simulink model "full_maneuver_single_veh"  (R2020a)
settings: Solver=VariableStepAuto  StartTime=0.0  StopTime=90  FixedStep=0.1  MaxStep=5e-2  RelTol=1e-3
InitFcn:
  | totalVehicles = 5;
  | if exist('vehStatesBus', 'var')==0
  | load vehBuses
  | end
  | if exist('vehErrorsBus', 'var')==0
  | load vehBuses
  | end
libraries: simulink x69, powerlib_meascontrol x6, autolibshared x6, dspsigops x3, eeGeneralControl x2
(part 5 of 6)

== system full_maneuver_single_veh/Lo/Regular Vehicle Following/switch ==
  errors : Inport
  errorsDot : Inport  Port=2
  gap : Inport  Port=3
  h : Inport  Port=4
  d0 : Inport  Port=5
  vRef : Inport  Port=6
  Compare To Constant : simulink/Logic and Bit Operations/Compare To Constant  relop=<=  const=0  OutDataTypeStr=boolean
  Demux1 : Demux  Outputs=2
  Gain1 : Gain
  MATLAB Function : MATLAB Function  TreatAsAtomicUnit=on
  Scope : Scope  NumInputPorts=2
  Selector : Selector  InputPortWidth=2  IndexOptions=Index vector (dialog)  Indices=[2]  OutputSizes=1
  Sum2 : Sum  Inputs=+-
  inRange : Outport  VectorParamsAs1DForOutWhenUnconnected=off
  wires:
  Demux1/2 -> MATLAB Function/6(ea)
  Demux1/1 -> MATLAB Function/5(ehDot)
  errorsDot/1 -> Demux1/1
  MATLAB Function/1(maxGap) -> Sum2/2, Scope/2
  Gain1/1 -> MATLAB Function/1(h)
  Compare To Constant/1 -> inRange/1
  Selector/1 -> MATLAB Function/4(ev)
  Sum2/1 -> Compare To Constant/1
  gap/1 -> Sum2/1, Scope/1
  errors/1 -> Selector/1
  h/1 -> Gain1/1
  vRef/1 -> MATLAB Function/3(vRef)
  d0/1 -> MATLAB Function/2(d0)

== system full_maneuver_single_veh/Lo/findLeader/Subsystem ==
  ego : Inport
  all : Inport  Port=2
  Enable : EnablePort
  MATLAB Function : MATLAB Function  TreatAsAtomicUnit=on
  idx : Outport  InitialOutput=1  VectorParamsAs1DForOutWhenUnconnected=off
  wires:
  ego/1 -> MATLAB Function/1(ego)
  MATLAB Function/1(leaderIdx) -> idx/1
  all/1 -> MATLAB Function/2(allVehicles)

== system full_maneuver_single_veh/Lo/findLeader/farAwayVeh ==
  ego : Inport  OutDataTypeStr=Bus: vehStatesBus
  Bus Assignment : BusAssignment  AssignedSignals=X
  Bus Selector : BusSelector  OutputSignals=X
  Constant : Constant  Value=1000
  Sum : Sum  Inputs=|++
  Out1 : Outport  OutDataTypeStr=Bus: vehStatesBus  VectorParamsAs1DForOutWhenUnconnected=off
  wires:
  Sum/1 -> Bus Assignment/2  "X"
  Bus Selector/1 -> Sum/1  "<X>"
  Bus Assignment/1 -> Out1/1
  Constant/1 -> Sum/2
  ego/1 -> Bus Selector/1, Bus Assignment/1

== system full_maneuver_single_veh/p1/Find Leader/Subsystem ==
  ego : Inport
  all : Inport  Port=2
  Enable : EnablePort
  MATLAB Function : MATLAB Function  TreatAsAtomicUnit=on
  idx : Outport  InitialOutput=1  VectorParamsAs1DForOutWhenUnconnected=off
  wires:
  ego/1 -> MATLAB Function/1(ego)
  MATLAB Function/1(leaderIdx) -> idx/1
  all/1 -> MATLAB Function/2(allVehicles)

== system full_maneuver_single_veh/p1/Find Leader/farAwayVeh ==
  ego : Inport  OutDataTypeStr=Bus: vehStatesBus
  Bus Assignment : BusAssignment  AssignedSignals=X
  Bus Selector : BusSelector  OutputSignals=X
  Constant : Constant  Value=1000
  Sum : Sum  Inputs=|++
  Out1 : Outport  OutDataTypeStr=Bus: vehStatesBus  VectorParamsAs1DForOutWhenUnconnected=off
  wires:
  ego/1 -> Bus Assignment/1, Bus Selector/1
  Constant/1 -> Sum/2
  Bus Assignment/1 -> Out1/1
  Bus Selector/1 -> Sum/1  "<X>"
  Sum/1 -> Bus Assignment/2  "X"

== system full_maneuver_single_veh/p1/Lateral Control/Full State Observer ==
  note: yhat
  note: xhat
  measuredOutputs : Inport
  delta : Inport  Port=2
  Add1 : Sum  Inputs=|-+
  Gain : Gain  Gain=B  Multiplication=Matrix(K*u)
  Gain1 : Gain  Gain=C  Multiplication=Matrix(K*u)
  Gain2 : Gain  Gain=L  Multiplication=Matrix(K*u)
  Gain3 : Gain  Gain=A  Multiplication=Matrix(K*u)
  Integrator : Integrator  InitialCondition=[y0; 0; 0; 0]
  Signal Specification : SignalSpecification  Dimensions=[size(C,1) 1]
  Sum : Sum  Inputs=+++
  xhat : Outport  VectorParamsAs1DForOutWhenUnconnected=off
  wires:
  Gain2/1 -> Sum/1
  Signal Specification/1 -> Gain2/1
  Gain3/1 -> Sum/2
  Gain/1 -> Sum/3
  delta/1 -> Gain/1
  measuredOutputs/1 -> Add1/2
  Sum/1 -> Integrator/1
  Gain1/1 -> Add1/1
  Integrator/1 -> Gain1/1, Gain3/1, xhat/1
  Add1/1 -> Signal Specification/1

== system full_maneuver_single_veh/p1/Maneuver State/Triggered Subsystem ==
  Trigger : TriggerPort  VariantControl=Variant
  Constant : Constant  OutDataTypeStr=fixdt(1,16,0)
  Out1 : Outport  InitialOutput=0  VectorParamsAs1DForOutWhenUnconnected=off
  wires:
  Constant/1 -> Out1/1

== system full_maneuver_single_veh/p1/Maneuver State/Triggered Subsystem1 ==
  Trigger : TriggerPort  VariantControl=Variant
  Constant : Constant  Value=true  OutDataTypeStr=boolean
  Out1 : Outport  OutDataTypeStr=boolean  InitialOutput=0  VectorParamsAs1DForOutWhenUnconnected=off
  wires:
  Constant/1 -> Out1/1

== system full_maneuver_single_veh/p1/Maneuver State/safeErrors ==
  errors : Inport
  AND : Logic  Inputs=1  IconShape=distinctive  AllPortsSameDT=off  OutDataTypeStr=boolean
  Compare To Constant4 : simulink/Logic and Bit Operations/Compare To Constant  relop=>=  const=-0.1  OutDataTypeStr=boolean
  Memory : Memory
  Triggered Subsystem1 : Subsystem  TreatAsAtomicUnit=on
  safetyFlag : Outport  VectorParamsAs1DForOutWhenUnconnected=off
  wires:
  Compare To Constant4/1 -> AND/1
  AND/1 -> Triggered Subsystem1/Trigger
  errors/1 -> Compare To Constant4/1
  Triggered Subsystem1/1(Out1) -> Memory/1
  Memory/1 -> safetyFlag/1

== system full_maneuver_single_veh/p1/Maneuver State/safeErrors1 ==
  errors : Inport
  AND : Logic  Inputs=1  IconShape=distinctive  AllPortsSameDT=off  OutDataTypeStr=boolean
  Compare To Constant4 : simulink/Logic and Bit Operations/Compare To Constant  relop=>=  const=-0.1  OutDataTypeStr=boolean
  safetyFlag : Outport  VectorParamsAs1DForOutWhenUnconnected=off
  wires:
  Compare To Constant4/1 -> AND/1
  errors/1 -> Compare To Constant4/1
  AND/1 -> safetyFlag/1

== system full_maneuver_single_veh/p1/Maneuver State/safeErrors2 ==
  errors : Inport
  AND : Logic  Inputs=1  IconShape=distinctive  AllPortsSameDT=off  OutDataTypeStr=boolean
  Compare To Constant4 : simulink/Logic and Bit Operations/Compare To Constant  relop=>=  const=-0.1  OutDataTypeStr=boolean
  safetyFlag : Outport  VectorParamsAs1DForOutWhenUnconnected=off
  wires:
  Compare To Constant4/1 -> AND/1
  AND/1 -> safetyFlag/1
  errors/1 -> Compare To Constant4/1

== system full_maneuver_single_veh/p1/Maneuver State/steadyState ==
  u : Inport
  AND : Logic  Inputs=1  IconShape=distinctive  AllPortsSameDT=off  OutDataTypeStr=boolean
  Abs2 : Abs
  Compare To Constant2 : simulink/Logic and Bit Operations/Compare To Constant  relop=<=  const=0.2  OutDataTypeStr=boolean
  Mux : Mux  Inputs=2
  Transport Delay2 : TransportDelay
  ssFlag : Outport  VectorParamsAs1DForOutWhenUnconnected=off
  wires:
  Compare To Constant2/1 -> AND/1
  u/1 -> Transport Delay2/1, Mux/2
  Abs2/1 -> Compare To Constant2/1
  Transport Delay2/1 -> Mux/1
  AND/1 -> ssFlag/1
  Mux/1 -> Abs2/1

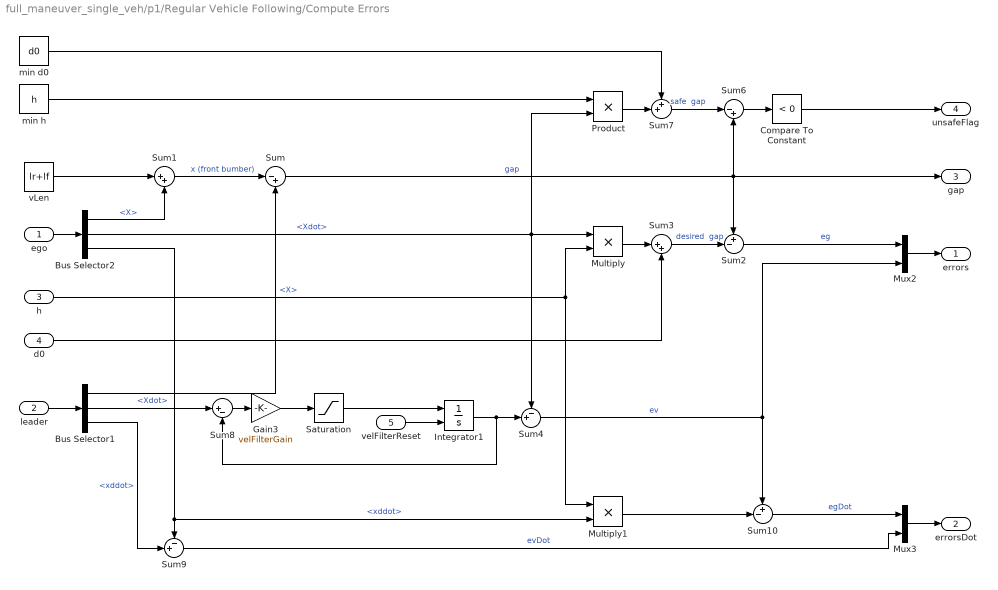
== system full_maneuver_single_veh/p1/Regular Vehicle Following/Compute Errors ==
  ego : Inport
  leader : Inport  Port=2
  h : Inport  Port=3
  d0 : Inport  Port=4
  velFilterReset : Inport  Port=5
  Bus Selector1 : BusSelector  OutputSignals=X,Xdot,xddot
  Bus Selector2 : BusSelector  OutputSignals=X,Xdot,xddot
  Compare To Constant : simulink/Logic and Bit Operations/Compare To Constant  relop=<  const=0  OutDataTypeStr=boolean
  Gain3 : Gain  Gain=velFilterGain
  Integrator1 : Integrator  ExternalReset=rising  InitialCondition=vx0
  Multiply : Product
  Multiply1 : Product
  Mux2 : Mux  Inputs=2
  Mux3 : Mux  Inputs=2
  Product : Product
  Saturation : Saturate  UpperLimit=maxAcceleration  LowerLimit=minAcceleration
  Sum : Sum  Inputs=|-+
  Sum1 : Sum  Inputs=|++
  Sum10 : Sum  Inputs=+-|
  Sum2 : Sum  Inputs=+-|
  Sum3 : Sum  Inputs=|++
  Sum4 : Sum  Inputs=-+|
  Sum6 : Sum  Inputs=|-+
  Sum7 : Sum  Inputs=++|
  Sum8 : Sum  Inputs=|+-
  Sum9 : Sum  Inputs=-+|
  min d0 : Constant  Value=d0
  min h : Constant  Value=h
  vLen : Constant  Value=lr+lf
  errors : Outport  VectorParamsAs1DForOutWhenUnconnected=off
  errorsDot : Outport  Port=2
  "gap " : Outport  Port=3  VectorParamsAs1DForOutWhenUnconnected=off
  unsafeFlag : Outport  Port=4  VectorParamsAs1DForOutWhenUnconnected=off
  wires:
  leader/1 -> Bus Selector1/1
  ego/1 -> Bus Selector2/1
  Mux3/1 -> errorsDot/1
  Sum9/1 -> Mux3/2  "evDot"
  Sum10/1 -> Mux3/1  "egDot"
  Multiply1/1 -> Sum10/2
  Bus Selector2/3 -> Multiply1/2, Sum9/1  "<xddot>"
  Bus Selector1/3 -> Sum9/2  "<xddot>"
  Sum8/1 -> Gain3/1
  Integrator1/1 -> Sum8/2, Sum4/2
  Saturation/1 -> Integrator1/1
  Gain3/1 -> Saturation/1
  Sum4/1 -> Sum10/1, Mux2/2  "ev"
  Bus Selector1/2 -> Sum8/1  "<Xdot>"
  h/1 -> Multiply1/1, Multiply/2
  Bus Selector2/1 -> Sum1/2  "<X>"
  Sum/1 -> "gap "/1, Sum6/2, Sum2/1  "gap"
  Multiply/1 -> Sum3/1
  min d0/1 -> Sum7/1
  vLen/1 -> Sum1/1
  d0/1 -> Sum3/2
  Bus Selector2/2 -> Product/2, Multiply/1, Sum4/1  "<Xdot>"
  Sum1/1 -> Sum/1  "x (front bumber)"
  Sum3/1 -> Sum2/2  "desired  gap"
  Product/1 -> Sum7/2
  Bus Selector1/1 -> Sum/2  "<X>"
  Sum2/1 -> Mux2/1  "eg"
  Compare To Constant/1 -> unsafeFlag/1
  min h/1 -> Product/1
  Sum7/1 -> Sum6/1  "safe  gap"
  Sum6/1 -> Compare To Constant/1
  velFilterReset/1 -> Integrator1/2
  Mux2/1 -> errors/1

== system full_maneuver_single_veh/p1/Regular Vehicle Following/Define Desired Distance ==
  extraSpaceFlag : Inport
  Constant : Constant  Value=h
  Constant1 : Constant  Value=d0
  Constant2 : Constant  Value=hLC
  Constant3 : Constant  Value=d0LC
  Demux : Demux  Outputs=2
  Integrator : Integrator  InitialCondition=[h d0]
  Mux : Mux  Inputs=2
  Mux1 : Mux  Inputs=2
  Saturation1 : Saturate  UpperLimit=hFilterSaturation/2  LowerLimit=-hFilterSaturation
  Sum5 : Sum  Inputs=|+-
  Switch : Switch  Criteria=u2 > Threshold
  hFilterGain : Gain  Gain=hFilterGain
  h : Outport
  d0 : Outport  Port=2
  wires:
  Demux/2 -> d0/1
  Demux/1 -> h/1
  Integrator/1 -> Sum5/2, Demux/1
  Saturation1/1 -> Integrator/1
  extraSpaceFlag/1 -> Switch/2
  Constant1/1 -> Mux/2
  Constant3/1 -> Mux1/2
  Switch/1 -> Sum5/1
  Mux1/1 -> Switch/1
  Sum5/1 -> hFilterGain/1
  Constant2/1 -> Mux1/1
  hFilterGain/1 -> Saturation1/1
  Constant/1 -> Mux/1
  Mux/1 -> Switch/3

== system full_maneuver_single_veh/p1/Regular Vehicle Following/Veh Following ==
  errors : Inport
  errorsDot : Inport  Port=2
  realInput : Inport  Port=3
  leaderChange : Inport  Port=4
  inRange : Inport  Port=5
  Demux : Demux  Outputs=2
  Demux1 : Demux  Outputs=2
  Gain : Gain  Gain=Ka
  Gain1 : Gain  Gain=Kdd
  Gain3 : Gain  Commented=on  Gain=10
  Integrator1 : Integrator  Commented=on  ExternalReset=either  InitialConditionSource=external  InitialCondition=vx0
  Kd : Gain  Gain=Kd
  Kp : Gain  Gain=Kp
  Saturation : Saturate  Commented=on  UpperLimit=maxComfAccel  LowerLimit=minAcceleration
  Saturation1 : Saturate  UpperLimit=maxGapError  LowerLimit=minGapError
  Scope : Scope  NumInputPorts=6
  Sum : Sum  Inputs=+-|
  Sum1 : Sum  Inputs=+++++
  Sum8 : Sum  Commented=on  Inputs=|+-
  Transport Delay : TransportDelay  DelayTime=0.1
  integralTerm : Subsystem
  u : Outport  VectorParamsAs1DForOutWhenUnconnected=off
  wires:
  Demux1/2 -> Gain/1  "evDot"
  Demux1/1 -> Gain1/1  "egDot"
  errorsDot/1 -> Demux1/1
  Sum1/1 -> u/1, Scope/6, Sum/1, Sum8/1
  Gain/1 -> Scope/5, Sum1/5
  Gain1/1 -> Scope/4, Sum1/4
  integralTerm/1(Out1) -> Transport Delay/1
  Sum/1 -> integralTerm/2(inputDiff)
  realInput/1 -> Integrator1/3, Sum/2
  Transport Delay/1 -> Scope/1, Sum1/1
  leaderChange/1 -> integralTerm/3(leaderChange)
  Demux/1 -> Saturation1/1  "eg"
  Kd/1 -> Scope/3, Sum1/3
  Demux/2 -> Kd/1  "ev"
  Saturation1/1 -> Kp/1, integralTerm/1(eh)
  errors/1 -> Demux/1
  Integrator1/1 -> Sum8/2
  Saturation/1 -> Integrator1/1
  Sum8/1 -> Gain3/1
  Gain3/1 -> Saturation/1
  Kp/1 -> Scope/2, Sum1/2
  inRange/1 -> Integrator1/2, integralTerm/Enable

== system full_maneuver_single_veh/p1/Regular Vehicle Following/Velocity Control ==
  ev : Inport
  ea : Inport  Port=2
  realInput : Inport  Port=3
  Abs : Abs
  Compare To Constant : simulink/Logic and Bit Operations/Compare To Constant  relop=<=  const=0.2  OutDataTypeStr=boolean
  Gain : Gain  Gain=velKd
  Scope : Scope  NumInputPorts=4
  Sum1 : Sum  Inputs=|-+
  Sum3 : Sum  Inputs=+++
  Transport Delay : TransportDelay  DelayTime=0.1
  integral term : Subsystem
  velKp : Gain  Gain=velKp
  u : Outport  VectorParamsAs1DForOutWhenUnconnected=off
  wires:
  Transport Delay/1 -> Sum1/2
  Compare To Constant/1 -> integral term/Enable
  integral term/1(Out1) -> Sum3/1, Scope/1
  Abs/1 -> Compare To Constant/1
  Sum1/1 -> Abs/1
  ev/1 -> velKp/1, integral term/1(ev)
  velKp/1 -> Scope/2, Sum3/2
  realInput/1 -> Sum1/1
  ea/1 -> Gain/1
  Gain/1 -> Scope/3, Sum3/3
  Sum3/1 -> u/1, Scope/4, Transport Delay/1

== system full_maneuver_single_veh/p1/Regular Vehicle Following/Velocity Error ==
  ego : Inport
  velRef : Inport  Port=2
  filterReset : Inport  Port=3
  Bus Selector : BusSelector  OutputSignals=Xdot,xddot
  Gain : Gain  Gain=-1
  Gain3 : Gain  Gain=velFilterGain
  Integrator1 : Integrator  ExternalReset=rising  InitialCondition=vx0
  NOT : Logic  Operator=NOT  IconShape=distinctive  AllPortsSameDT=off  OutDataTypeStr=boolean
  Saturation : Saturate  UpperLimit=maxComfAccel  LowerLimit=minComfAccel
  Sum : Sum  Inputs=+-|
  Sum8 : Sum  Inputs=|+-
  ev : Outport
  ea : Outport  Port=2
  wires:
  Sum8/1 -> Gain3/1
  Gain3/1 -> Saturation/1
  Saturation/1 -> Integrator1/1
  velRef/1 -> Sum8/1
  Integrator1/1 -> Sum/1, Sum8/2
  ego/1 -> Bus Selector/1
  Bus Selector/1 -> Sum/2  "<Xdot>"
  Bus Selector/2 -> Gain/1  "<xddot>"
  Sum/1 -> ev/1
  Gain/1 -> ea/1
  filterReset/1 -> NOT/1
  NOT/1 -> Integrator1/2

== system full_maneuver_single_veh/p1/Regular Vehicle Following/switch free flow ==
  errors : Inport
  errorsDot : Inport  Port=2
  gap : Inport  Port=3
  h : Inport  Port=4
  d0 : Inport  Port=5
  vRef : Inport  Port=6
  Demux1 : Demux  Outputs=2
  Gain1 : Gain
  MATLAB Function : MATLAB Function  TreatAsAtomicUnit=on
  Relay : Relay  OnSwitchValue=1  OffSwitchValue=-1
  Scope : Scope  NumInputPorts=2
  Selector : Selector  InputPortWidth=2  IndexOptions=Index vector (dialog)  Indices=[2]  OutputSizes=1
  Sum2 : Sum  Inputs=-+
  inRange : Outport  VectorParamsAs1DForOutWhenUnconnected=off
  wires:
  Demux1/2 -> MATLAB Function/6(ea)
  Demux1/1 -> MATLAB Function/5(ehDot)
  errorsDot/1 -> Demux1/1
  MATLAB Function/1(maxGap) -> Sum2/2, Scope/2
  Gain1/1 -> MATLAB Function/1(h)
  Relay/1 -> inRange/1
  Selector/1 -> MATLAB Function/4(ev)
  Sum2/1 -> Relay/1
  gap/1 -> Sum2/1, Scope/1
  errors/1 -> Selector/1
  h/1 -> Gain1/1
  vRef/1 -> MATLAB Function/3(vRef)
  d0/1 -> MATLAB Function/2(d0)

== system full_maneuver_single_veh/p1/Virtual Vehicle Following/Compute Errors ==
  ego : Inport
  leader : Inport  Port=2
  h : Inport  Port=3
  d0 : Inport  Port=4
  velFilterReset : Inport  Port=5
  Bus Selector1 : BusSelector  OutputSignals=X,Xdot,xddot
  Bus Selector2 : BusSelector  OutputSignals=X,Xdot,xddot
  Compare To Constant : simulink/Logic and Bit Operations/Compare To Constant  relop=<  const=0  OutDataTypeStr=boolean
  Gain3 : Gain  Gain=velFilterGain
  Integrator1 : Integrator  ExternalReset=rising  InitialCondition=vx0
  Multiply : Product
  Multiply1 : Product
  Mux2 : Mux  Inputs=2
  Mux3 : Mux  Inputs=2
  Product : Product
  Saturation : Saturate  UpperLimit=maxAcceleration  LowerLimit=minAcceleration
  Sum : Sum  Inputs=|-+
  Sum1 : Sum  Inputs=|++
  Sum10 : Sum  Inputs=+-|
  Sum2 : Sum  Inputs=+-|
  Sum3 : Sum  Inputs=|++
  Sum4 : Sum  Inputs=-+|
  Sum6 : Sum  Inputs=|-+
  Sum7 : Sum  Inputs=++|
  Sum8 : Sum  Inputs=|+-
  Sum9 : Sum  Inputs=-+|
  min d0 : Constant  Value=d0
  min h : Constant  Value=h
  vLen : Constant  Value=lr+lf
  errors : Outport  VectorParamsAs1DForOutWhenUnconnected=off
  errorsDot : Outport  Port=2
  "gap " : Outport  Port=3  VectorParamsAs1DForOutWhenUnconnected=off
  unsafeFlag : Outport  Port=4  VectorParamsAs1DForOutWhenUnconnected=off
  wires:
  leader/1 -> Bus Selector1/1
  ego/1 -> Bus Selector2/1
  Mux3/1 -> errorsDot/1
  Sum9/1 -> Mux3/2  "evDot"
  Sum10/1 -> Mux3/1  "egDot"
  Multiply1/1 -> Sum10/2
  Bus Selector2/3 -> Multiply1/2, Sum9/1  "<xddot>"
  Bus Selector1/3 -> Sum9/2  "<xddot>"
  Sum8/1 -> Gain3/1
  Integrator1/1 -> Sum8/2, Sum4/2
  Saturation/1 -> Integrator1/1
  Gain3/1 -> Saturation/1
  Sum4/1 -> Sum10/1, Mux2/2  "ev"
  Bus Selector1/2 -> Sum8/1  "<Xdot>"
  h/1 -> Multiply1/1, Multiply/2
  Bus Selector2/1 -> Sum1/2  "<X>"
  Sum/1 -> Sum6/2, "gap "/1, Sum2/1  "gap"
  Multiply/1 -> Sum3/1
  min d0/1 -> Sum7/1
  vLen/1 -> Sum1/1
  d0/1 -> Sum3/2
  Bus Selector2/2 -> Product/2, Multiply/1, Sum4/1  "<Xdot>"
  Sum1/1 -> Sum/1  "x (front bumber)"
  Sum3/1 -> Sum2/2  "desired  gap"
  Product/1 -> Sum7/2
  Bus Selector1/1 -> Sum/2  "<X>"
  Sum2/1 -> Mux2/1  "eg"
  Compare To Constant/1 -> unsafeFlag/1
  min h/1 -> Product/1
  Sum7/1 -> Sum6/1  "safe  gap"
  Sum6/1 -> Compare To Constant/1
  velFilterReset/1 -> Integrator1/2
  Mux2/1 -> errors/1

== system full_maneuver_single_veh/p1/Virtual Vehicle Following/Define Desired Distance ==
  extraSpaceFlag : Inport
  Constant : Constant  Value=h
  Constant1 : Constant  Value=d0
  Constant2 : Constant  Value=hLC
  Constant3 : Constant  Value=d0LC
  Demux : Demux  Outputs=2
  Integrator : Integrator  InitialCondition=[h d0]
  Mux : Mux  Inputs=2
  Mux1 : Mux  Inputs=2
  Saturation1 : Saturate  UpperLimit=hFilterSaturation/2  LowerLimit=-hFilterSaturation
  Sum5 : Sum  Inputs=|+-
  Switch : Switch  Criteria=u2 > Threshold
  hFilterGain : Gain  Gain=hFilterGain
  h : Outport
  d0 : Outport  Port=2
  wires:
  Demux/2 -> d0/1
  Demux/1 -> h/1
  Integrator/1 -> Sum5/2, Demux/1
  Saturation1/1 -> Integrator/1
  extraSpaceFlag/1 -> Switch/2
  Constant1/1 -> Mux/2
  Constant3/1 -> Mux1/2
  Switch/1 -> Sum5/1
  Mux1/1 -> Switch/1
  Sum5/1 -> hFilterGain/1
  Constant2/1 -> Mux1/1
  hFilterGain/1 -> Saturation1/1
  Constant/1 -> Mux/1
  Mux/1 -> Switch/3

== system full_maneuver_single_veh/p1/Virtual Vehicle Following/Min Velocity Control ==
  ev : Inport
  ea : Inport  Port=2
  realInput : Inport  Port=3
  Abs : Abs
  Compare To Constant : simulink/Logic and Bit Operations/Compare To Constant  relop=<=  const=0.2  OutDataTypeStr=boolean
  Gain : Gain  Gain=velKd
  Scope : Scope  NumInputPorts=4
  Sum1 : Sum  Inputs=|-+
  Sum3 : Sum  Inputs=+++
  Transport Delay : TransportDelay  DelayTime=0.1
  integral term : Subsystem
  velKp : Gain  Gain=velKp
  u : Outport  VectorParamsAs1DForOutWhenUnconnected=off
  wires:
  Transport Delay/1 -> Sum1/2
  Compare To Constant/1 -> integral term/Enable
  integral term/1(Out1) -> Sum3/1, Scope/1
  Abs/1 -> Compare To Constant/1
  Sum1/1 -> Abs/1
  ev/1 -> velKp/1, integral term/1(ev)
  velKp/1 -> Scope/2, Sum3/2
  Sum3/1 -> Scope/4, Transport Delay/1, u/1
  realInput/1 -> Sum1/1
  ea/1 -> Gain/1
  Gain/1 -> Scope/3, Sum3/3

== system full_maneuver_single_veh/p1/Virtual Vehicle Following/Min Velocity Error ==
  ego : Inport
  velRef : Inport  Port=2
  filterReset : Inport  Port=3
  Bus Selector : BusSelector  OutputSignals=Xdot,xddot
  Gain : Gain  Gain=-1
  Gain3 : Gain  Gain=velFilterGain
  Integrator1 : Integrator  ExternalReset=rising  InitialCondition=vx0
  Saturation : Saturate  UpperLimit=maxComfAccel  LowerLimit=minComfAccel
  Sum : Sum  Inputs=+-|
  Sum8 : Sum  Inputs=|+-
  ev : Outport
  ea : Outport  Port=2
  wires:
  filterReset/1 -> Integrator1/2
  Gain/1 -> ea/1
  Sum/1 -> ev/1
  Bus Selector/2 -> Gain/1  "<xddot>"
  Bus Selector/1 -> Sum/2  "<Xdot>"
  ego/1 -> Bus Selector/1
  Integrator1/1 -> Sum8/2, Sum/1
  velRef/1 -> Sum8/1
  Saturation/1 -> Integrator1/1
  Gain3/1 -> Saturation/1
  Sum8/1 -> Gain3/1

== system full_maneuver_single_veh/p1/Virtual Vehicle Following/Virtual Leader Following ==
  errors : Inport
  errorsDot : Inport  Port=2
  realInput : Inport  Port=3
  leaderChange : Inport  Port=4
  inRange : Inport  Port=5
  Demux : Demux  Outputs=2
  Demux1 : Demux  Outputs=2
  Gain : Gain  Gain=10
  Gain3 : Gain  Gain=Ka
  Gain4 : Gain  Gain=Kdd
  Gain5 : Gain  Gain=10
  Integrator1 : Integrator  ExternalReset=rising  InitialConditionSource=external  InitialCondition=vx0
  Integrator2 : Integrator  ExternalReset=rising
  Kd : Gain  Gain=Kd
  Kp : Gain  Gain=Kp
  Saturation : Saturate  UpperLimit=maxComfAccel  LowerLimit=minAcceleration
  Saturation1 : Saturate  UpperLimit=maxGapError  LowerLimit=-maxGapError*2
  Scope : Scope  NumInputPorts=6
  Sum : Sum  Inputs=+-|
  Sum1 : Sum  Inputs=+++++
  Sum8 : Sum  Inputs=|+-
  Sum9 : Sum  Inputs=|+-
  Transport Delay : TransportDelay  DelayTime=0.1
  integralTerm : Subsystem
  u : Outport  VectorParamsAs1DForOutWhenUnconnected=off
  wires:
  errorsDot/1 -> Demux1/1
  errors/1 -> Demux/1
  Saturation1/1 -> Sum9/1
  Sum9/1 -> Gain/1
  Gain/1 -> Integrator2/1
  Demux/1 -> Saturation1/1
  Kd/1 -> Scope/3, Sum1/3
  Gain5/1 -> Saturation/1
  inRange/1 -> integralTerm/Enable, Integrator1/2
  Transport Delay/1 -> Scope/1, Sum1/1
  Integrator2/1 -> integralTerm/1(eh), Kp/1, Sum9/2
  Kp/1 -> Scope/2, Sum1/2
  Sum/1 -> integralTerm/2(inputDiff)
  Sum8/1 -> Gain5/1
  realInput/1 -> Integrator1/3, Sum/2
  Gain4/1 -> Scope/4, Sum1/4
  Saturation/1 -> Integrator1/1
  Demux/2 -> Kd/1  "ev"
  Gain3/1 -> Scope/5, Sum1/5
  Integrator1/1 -> u/1, Sum8/2
  Sum1/1 -> Sum/1, Scope/6, Sum8/1
  integralTerm/1(Out1) -> Transport Delay/1
  leaderChange/1 -> Integrator2/2, integralTerm/3(leaderChange)
  Demux1/1 -> Gain4/1  "egDot"
  Demux1/2 -> Gain3/1  "evDot"

== system full_maneuver_single_veh/p1/Virtual Vehicle Following/switch min vel ==
  errors : Inport
  errorsDot : Inport  Port=2
  gap : Inport  Port=3
  h : Inport  Port=4
  d0 : Inport  Port=5
  vRef : Inport  Port=6
  Demux1 : Demux  Outputs=2
  Gain1 : Gain
  MATLAB Function : MATLAB Function  TreatAsAtomicUnit=on
  Relay1 : Relay  OnSwitchValue=1  OffSwitchValue=-1
  Scope : Scope  NumInputPorts=2
  Scope1 : Scope  NumInputPorts=2
  Selector : Selector  InputPortWidth=2  IndexOptions=Index vector (dialog)  Indices=[2]  OutputSizes=1
  Sum2 : Sum  Inputs=-+
  inRange : Outport  VectorParamsAs1DForOutWhenUnconnected=off
  wires:
  Demux1/2 -> MATLAB Function/6(ea)
  Demux1/1 -> MATLAB Function/5(ehDot)
  errorsDot/1 -> Demux1/1
  MATLAB Function/1(maxGap) -> Sum2/2, Scope/2
  Gain1/1 -> MATLAB Function/1(h)
  Relay1/1 -> Scope1/2, inRange/1
  Selector/1 -> MATLAB Function/4(ev)
  Sum2/1 -> Relay1/1, Scope1/1
  gap/1 -> Sum2/1, Scope/1
  errors/1 -> Selector/1
  h/1 -> Gain1/1
  vRef/1 -> MATLAB Function/3(vRef)
  d0/1 -> MATLAB Function/2(d0)

== system full_maneuver_single_veh/Fd/Maneuver State/safeErrors/Triggered Subsystem1 ==
  Trigger : TriggerPort  VariantControl=Variant
  Constant : Constant  Value=true  OutDataTypeStr=boolean
  Out1 : Outport  OutDataTypeStr=boolean  InitialOutput=0  VectorParamsAs1DForOutWhenUnconnected=off
  wires:
  Constant/1 -> Out1/1

== system full_maneuver_single_veh/Fd/Regular Vehicle Following/Veh Following/integralTerm ==
  eh : Inport
  inputDiff : Inport  Port=2
  leaderChange : Inport  Port=3
  Enable : EnablePort  ShowOutputPort=on
  Anti-windup gain : Gain  Gain=sqrt(Ki/Kd)
  Integrator : Integrator  ExternalReset=either
  Ki : Gain  Gain=Ki
  Scope : Scope  NumInputPorts=2
  Sum5 : Sum  Inputs=-+|
  XOR : Logic  Operator=XOR  IconShape=distinctive  AllPortsSameDT=off  OutDataTypeStr=boolean
  Out1 : Outport  OutputWhenDisabled=reset  InitialOutput=0  VectorParamsAs1DForOutWhenUnconnected=off
  wires:
  eh/1 -> Ki/1
  Integrator/1 -> Out1/1
  XOR/1 -> Integrator/2
  leaderChange/1 -> XOR/1
  Enable/1 -> XOR/2
  Sum5/1 -> Integrator/1, Scope/2
  Ki/1 -> Sum5/2
  Anti-windup gain/1 -> Sum5/1, Scope/1
  inputDiff/1 -> Anti-windup gain/1

== system full_maneuver_single_veh/Fd/Regular Vehicle Following/Velocity Control/integral term ==
  ev : Inport
  Enable : EnablePort  StatesWhenEnabling=reset
  Integrator2 : Integrator
  velKi : Gain  Gain=velKi
  Out1 : Outport  OutputWhenDisabled=reset  InitialOutput=0
  wires:
  velKi/1 -> Integrator2/1
  Integrator2/1 -> Out1/1
  ev/1 -> velKi/1

== system full_maneuver_single_veh/Fd/Virtual Vehicle Following/Min Velocity Control/integral term ==
  ev : Inport
  Enable : EnablePort  StatesWhenEnabling=reset
  Integrator2 : Integrator
  velKi : Gain  Gain=velKi
  Out1 : Outport  OutputWhenDisabled=reset  InitialOutput=0
  wires:
  velKi/1 -> Integrator2/1
  Integrator2/1 -> Out1/1
  ev/1 -> velKi/1

== system full_maneuver_single_veh/Fd/Virtual Vehicle Following/Virtual Leader Following/integralTerm ==
  eh : Inport
  inputDiff : Inport  Port=2
  leaderChange : Inport  Port=3
  Enable : EnablePort  ShowOutputPort=on
  Anti-windup gain : Gain  Gain=sqrt(Ki/Kd)
  Integrator : Integrator  ExternalReset=either
  Ki : Gain  Gain=Ki
  Scope : Scope  NumInputPorts=2
  Sum5 : Sum  Inputs=-+|
  XOR : Logic  Operator=XOR  IconShape=distinctive  AllPortsSameDT=off  OutDataTypeStr=boolean
  Out1 : Outport  OutputWhenDisabled=reset  InitialOutput=0  VectorParamsAs1DForOutWhenUnconnected=off
  wires:
  eh/1 -> Ki/1
  Integrator/1 -> Out1/1
  XOR/1 -> Integrator/2
  leaderChange/1 -> XOR/1
  Enable/1 -> XOR/2
  Sum5/1 -> Integrator/1, Scope/2
  Ki/1 -> Sum5/2
  Anti-windup gain/1 -> Sum5/1, Scope/1
  inputDiff/1 -> Anti-windup gain/1

== system full_maneuver_single_veh/Fd_bkp/Maneuver State/safeErrors/Triggered Subsystem1 ==
  Trigger : TriggerPort  VariantControl=Variant
  Constant : Constant  Value=true  OutDataTypeStr=boolean
  Out1 : Outport  OutDataTypeStr=boolean  InitialOutput=0  VectorParamsAs1DForOutWhenUnconnected=off
  wires:
  Constant/1 -> Out1/1

== system full_maneuver_single_veh/Fd_bkp/Regular Vehicle Following/Veh Following/integralTerm ==
  eh : Inport
  leaderChange : Inport  Port=2
  inputDiff : Inport  Port=3
  Enable : EnablePort  ShowOutputPort=on
  Anti-windup gain : Gain  Gain=sqrt(Ki/Kd)
  Integrator : Integrator  ExternalReset=rising
  Ki : Gain  Gain=Ki
  Sum5 : Sum  Inputs=-+|
  XOR : Logic  Operator=XOR  IconShape=distinctive  AllPortsSameDT=off  OutDataTypeStr=boolean
  Out1 : Outport  OutputWhenDisabled=reset  InitialOutput=0  VectorParamsAs1DForOutWhenUnconnected=off
  wires:
  eh/1 -> Ki/1
  Integrator/1 -> Out1/1
  XOR/1 -> Integrator/2
  leaderChange/1 -> XOR/1
  Enable/1 -> XOR/2
  Sum5/1 -> Integrator/1
  Ki/1 -> Sum5/2
  Anti-windup gain/1 -> Sum5/1
  inputDiff/1 -> Anti-windup gain/1

== system full_maneuver_single_veh/Fd_bkp/Regular Vehicle Following/Velocity Control/integral term ==
  ev : Inport
  Enable : EnablePort  StatesWhenEnabling=reset
  Integrator2 : Integrator
  velKi : Gain  Gain=velKi
  Out1 : Outport  OutputWhenDisabled=reset  InitialOutput=0
  wires:
  velKi/1 -> Integrator2/1
  Integrator2/1 -> Out1/1
  ev/1 -> velKi/1

== system full_maneuver_single_veh/Fd_bkp/Virtual Vehicle Following/Velocity Control1/integral term ==
  ev : Inport
  Enable : EnablePort  StatesWhenEnabling=reset
  Integrator2 : Integrator
  velKi : Gain  Gain=velKi
  Out1 : Outport  OutputWhenDisabled=reset  InitialOutput=0
  wires:
  velKi/1 -> Integrator2/1
  Integrator2/1 -> Out1/1
  ev/1 -> velKi/1

== system full_maneuver_single_veh/Fd_bkp/Virtual Vehicle Following/Velocity Control2/integral term ==
  ev : Inport
  Enable : EnablePort  StatesWhenEnabling=reset
  Integrator2 : Integrator
  velKi : Gain  Gain=velKi
  Out1 : Outport  OutputWhenDisabled=reset  InitialOutput=0
  wires:
  ev/1 -> velKi/1
  Integrator2/1 -> Out1/1
  velKi/1 -> Integrator2/1

== system full_maneuver_single_veh/Fd_bkp/Virtual Vehicle Following/Virtual Leader Following/integralTerm ==
  eh : Inport
  leaderChange : Inport  Port=2
  inputDiff : Inport  Port=3
  Enable : EnablePort  ShowOutputPort=on
  Anti-windup gain : Gain  Gain=sqrt(Ki/Kd)
  Integrator : Integrator  ExternalReset=rising
  Ki : Gain  Gain=Ki
  Sum5 : Sum  Inputs=-+|
  XOR : Logic  Operator=XOR  IconShape=distinctive  AllPortsSameDT=off  OutDataTypeStr=boolean
  Out1 : Outport  OutputWhenDisabled=reset  InitialOutput=0  VectorParamsAs1DForOutWhenUnconnected=off
  wires:
  eh/1 -> Ki/1
  Integrator/1 -> Out1/1
  XOR/1 -> Integrator/2
  leaderChange/1 -> XOR/1
  Enable/1 -> XOR/2
  Sum5/1 -> Integrator/1
  Ki/1 -> Sum5/2
  Anti-windup gain/1 -> Sum5/1
  inputDiff/1 -> Anti-windup gain/1

== system full_maneuver_single_veh/Fo/Regular Vehicle Following/Veh Following/integralTerm ==
  eh : Inport
  inputDiff : Inport  Port=2
  leaderChange : Inport  Port=3
  Enable : EnablePort  ShowOutputPort=on
  Anti-windup gain : Gain  Gain=sqrt(Ki/Kd)
  Integrator : Integrator  ExternalReset=either
  Ki : Gain  Gain=Ki
  Sum5 : Sum  Inputs=-+|
  XOR : Logic  Operator=XOR  IconShape=distinctive  AllPortsSameDT=off  OutDataTypeStr=boolean
  Out1 : Outport  OutputWhenDisabled=reset  InitialOutput=0  VectorParamsAs1DForOutWhenUnconnected=off
  wires:
  eh/1 -> Ki/1
  Integrator/1 -> Out1/1
  XOR/1 -> Integrator/2
  leaderChange/1 -> XOR/1
  Enable/1 -> XOR/2
  Sum5/1 -> Integrator/1
  Ki/1 -> Sum5/2
  Anti-windup gain/1 -> Sum5/1
  inputDiff/1 -> Anti-windup gain/1

== system full_maneuver_single_veh/Fo/Regular Vehicle Following/Velocity Control/integral term ==
  ev : Inport
  Enable : EnablePort  StatesWhenEnabling=reset
  Integrator2 : Integrator
  velKi : Gain  Gain=velKi
  Out1 : Outport  OutputWhenDisabled=reset  InitialOutput=0
  wires:
  velKi/1 -> Integrator2/1
  Integrator2/1 -> Out1/1
  ev/1 -> velKi/1

== system full_maneuver_single_veh/Ld/Regular Vehicle Following/Veh Following/integralTerm ==
  eh : Inport
  inputDiff : Inport  Port=2
  leaderChange : Inport  Port=3
  Enable : EnablePort  ShowOutputPort=on
  Anti-windup gain : Gain  Gain=sqrt(Ki/Kd)
  Integrator : Integrator  ExternalReset=either
  Ki : Gain  Gain=Ki
  Sum5 : Sum  Inputs=-+|
  XOR : Logic  Operator=XOR  IconShape=distinctive  AllPortsSameDT=off  OutDataTypeStr=boolean
  Out1 : Outport  OutputWhenDisabled=reset  InitialOutput=0  VectorParamsAs1DForOutWhenUnconnected=off
  wires:
  eh/1 -> Ki/1
  Integrator/1 -> Out1/1
  XOR/1 -> Integrator/2
  leaderChange/1 -> XOR/1
  Enable/1 -> XOR/2
  Sum5/1 -> Integrator/1
  Ki/1 -> Sum5/2
  Anti-windup gain/1 -> Sum5/1
  inputDiff/1 -> Anti-windup gain/1

== system full_maneuver_single_veh/Ld/Regular Vehicle Following/Velocity Control/integral term ==
  ev : Inport
  Enable : EnablePort  StatesWhenEnabling=reset
  Integrator2 : Integrator
  velKi : Gain  Gain=velKi
  Out1 : Outport  OutputWhenDisabled=reset  InitialOutput=0
  wires:
  velKi/1 -> Integrator2/1
  Integrator2/1 -> Out1/1
  ev/1 -> velKi/1

== system full_maneuver_single_veh/Lo/Regular Vehicle Following/Veh Following/integralTerm ==
  eh : Inport
  inputDiff : Inport  Port=2
  leaderChange : Inport  Port=3
  Enable : EnablePort  ShowOutputPort=on
  Anti-windup gain : Gain  Gain=sqrt(Ki/Kd)
  Integrator : Integrator  ExternalReset=either
  Ki : Gain  Gain=Ki
  Sum5 : Sum  Inputs=-+|
  XOR : Logic  Operator=XOR  IconShape=distinctive  AllPortsSameDT=off  OutDataTypeStr=boolean
  Out1 : Outport  OutputWhenDisabled=reset  InitialOutput=0  VectorParamsAs1DForOutWhenUnconnected=off
  wires:
  inputDiff/1 -> Anti-windup gain/1
  Anti-windup gain/1 -> Sum5/1
  Ki/1 -> Sum5/2
  Sum5/1 -> Integrator/1
  Enable/1 -> XOR/2
  leaderChange/1 -> XOR/1
  XOR/1 -> Integrator/2
  Integrator/1 -> Out1/1
  eh/1 -> Ki/1

== system full_maneuver_single_veh/Lo/Regular Vehicle Following/Velocity Control/integral term ==
  ev : Inport
  Enable : EnablePort  StatesWhenEnabling=reset
  Integrator2 : Integrator
  velKi : Gain  Gain=velKi
  Out1 : Outport  OutputWhenDisabled=reset  InitialOutput=0
  wires:
  ev/1 -> velKi/1
  Integrator2/1 -> Out1/1
  velKi/1 -> Integrator2/1

== system full_maneuver_single_veh/p1/Maneuver State/safeErrors/Triggered Subsystem1 ==
  Trigger : TriggerPort  VariantControl=Variant
  Constant : Constant  Value=true  OutDataTypeStr=boolean
  Out1 : Outport  OutDataTypeStr=boolean  InitialOutput=0  VectorParamsAs1DForOutWhenUnconnected=off
  wires:
  Constant/1 -> Out1/1

== system full_maneuver_single_veh/p1/Regular Vehicle Following/Veh Following/integralTerm ==
  eh : Inport
  inputDiff : Inport  Port=2
  leaderChange : Inport  Port=3
  Enable : EnablePort  ShowOutputPort=on
  Anti-windup gain : Gain  Gain=sqrt(Ki/Kd)
  Integrator : Integrator  ExternalReset=either
  Ki : Gain  Gain=Ki
  Scope : Scope  NumInputPorts=2
  Sum5 : Sum  Inputs=-+|
  XOR : Logic  Operator=XOR  IconShape=distinctive  AllPortsSameDT=off  OutDataTypeStr=boolean
  Out1 : Outport  OutputWhenDisabled=reset  InitialOutput=0  VectorParamsAs1DForOutWhenUnconnected=off
  wires:
  inputDiff/1 -> Anti-windup gain/1
  Anti-windup gain/1 -> Scope/1, Sum5/1
  Ki/1 -> Sum5/2
  Sum5/1 -> Scope/2, Integrator/1
  Enable/1 -> XOR/2
  leaderChange/1 -> XOR/1
  XOR/1 -> Integrator/2
  Integrator/1 -> Out1/1
  eh/1 -> Ki/1

== system full_maneuver_single_veh/p1/Regular Vehicle Following/Velocity Control/integral term ==
  ev : Inport
  Enable : EnablePort  StatesWhenEnabling=reset
  Integrator2 : Integrator
  velKi : Gain  Gain=velKi
  Out1 : Outport  OutputWhenDisabled=reset  InitialOutput=0
  wires:
  ev/1 -> velKi/1
  Integrator2/1 -> Out1/1
  velKi/1 -> Integrator2/1

== system full_maneuver_single_veh/p1/Virtual Vehicle Following/Min Velocity Control/integral term ==
  ev : Inport
  Enable : EnablePort  StatesWhenEnabling=reset
  Integrator2 : Integrator
  velKi : Gain  Gain=velKi
  Out1 : Outport  OutputWhenDisabled=reset  InitialOutput=0
  wires:
  ev/1 -> velKi/1
  Integrator2/1 -> Out1/1
  velKi/1 -> Integrator2/1

== system full_maneuver_single_veh/p1/Virtual Vehicle Following/Virtual Leader Following/integralTerm ==
  eh : Inport
  inputDiff : Inport  Port=2
  leaderChange : Inport  Port=3
  Enable : EnablePort  ShowOutputPort=on
  Anti-windup gain : Gain  Gain=sqrt(Ki/Kd)
  Integrator : Integrator  ExternalReset=either
  Ki : Gain  Gain=Ki
  Scope : Scope  NumInputPorts=2
  Sum5 : Sum  Inputs=-+|
  XOR : Logic  Operator=XOR  IconShape=distinctive  AllPortsSameDT=off  OutDataTypeStr=boolean
  Out1 : Outport  OutputWhenDisabled=reset  InitialOutput=0  VectorParamsAs1DForOutWhenUnconnected=off
  wires:
  inputDiff/1 -> Anti-windup gain/1
  Anti-windup gain/1 -> Scope/1, Sum5/1
  Ki/1 -> Sum5/2
  Sum5/1 -> Scope/2, Integrator/1
  Enable/1 -> XOR/2
  leaderChange/1 -> XOR/1
  XOR/1 -> Integrator/2
  Integrator/1 -> Out1/1
  eh/1 -> Ki/1

== matlab function full_maneuver_single_veh/Fd_bkp/Regular Vehicle Following/switch free flow/MATLAB Function ==
  data: h input; maxGap output; d0 input; vRef input; ev input; ehDot input; ea input; Kp parameter; Kd parameter; Ka parameter; Kdd parameter
function maxGap = followingGapThreshold(h, d0, vRef, ev, ehDot, ea, Kp, Kd, Ka, Kdd)

maxGap = h*vRef + d0 - 1/Kp*(Kd*ev + Kdd*ehDot + Ka*ea);

== matlab function full_maneuver_single_veh/Fd_bkp/Virtual Follower Manager/determineVirtualFollower ==
  data: nVehicles input; posInPlatoon input; lcStrategy input; virtualFollowerIdx output
function virtualFollowerIdx  = ...
    determineVirtualFollower(nVehicles, posInPlatoon, lcStrategy)

% Important assumption:
% The array of vehicles is ordered as [Ld, Fd, Lo, p1, ..., pN, Fo]

% To consider: would it be more organized to have two vehicle arrays (one 
% for each lane)?

switch lcStrategy
    case {1, 2} % synchronous, leader changes first
        virtualFollowerIdx = 2;
    case 3 % last veh changes first
        if posInPlatoon == nVehicles-4
            virtualFollowerIdx = 2;
        else
            virtualFollowerIdx = 3 + (posInPlatoon + 1);
        end
    otherwise
        error('[determineVirtualFollower in Simulink model] Unknown lane changing strategy]')
end

end

== matlab function full_maneuver_single_veh/Fd_bkp/Virtual Leader Manager/determineVirtualLeader ==
  data: nVehicles input; lcFlag input; lcDone input; virtualLeaderIdx output; posInPlatoon input; lcStrategy input
function virtualLeaderIdx  = ...
    determineVirtualLeader(nVehicles, lcFlag, lcDone, posInPlatoon, lcStrategy)

% Important assumption:
% The array of vehicles is ordered as [Ld, Fd, Lo, p1, ..., pN, Fo]

% To consider: would it be more organized to have two vehicle arrays (one 
% for each lane)?

if ~lcFlag% gap generating vehicle
    virtualLeaderIdx = nVehicles-1; % last platoon vehicle
    
else % lane changing vehicle
    switch lcStrategy
        case {1, 2} % synchronous, leader changes first
            if posInPlatoon == 1
                virtualLeaderIdx = 1;
            else
                virtualLeaderIdx = 3 + (posInPlatoon - 1);
            end
            
        case 3 % last veh changes first
            if ~lcDone
                virtualLeaderIdx = 1;
            else
                if posInPlatoon == 1
                    virtualLeaderIdx = 1;
                else
                    virtualLeaderIdx = 3 + (posInPlatoon - 1);
                end
            end
            
        otherwise
            error('[determineVirtualLeader in Simulink model] Unknown lane changing strategy]')
    end
end

end

== stateflow chart full_maneuver_single_veh/Fd_bkp/Virtual Vehicle Following/Chart ==
  state SpeedControlFreeFlow
    entry:
    state=2;
    during:
    u = uFreeFlowVelControl;
  state VehFollowing
    entry:
    state=0;
    during:
    u = uVehFoll;
  state SpeedControlMin
    entry:
    state = 1;
    during:
    u = uMinVelControl;
  state LogicError
    entry:
    state=-1;
  (default) -> VehFollowing
  VehFollowing -> SpeedControlFreeFlow [order 2] : [~leaderInRange]
  SpeedControlFreeFlow -> VehFollowing [order 1] : [leaderInRange]
  VehFollowing -> SpeedControlMin [order 1] : [~leaderInRangeBehind]
  SpeedControlMin -> VehFollowing [order 1] : [leaderInRangeBehind]
  LogicError -> VehFollowing
  SpeedControlFreeFlow -> LogicError [order 2] : [~leaderInRangeBehind]
  SpeedControlMin -> LogicError [order 2] : [~leaderInRange]
  data: uVehFoll input size=1; leaderInRange input; leaderInRangeBehind input size=1; uFreeFlowVelControl input; state output size=1; u output size=1; uMinVelControl input double

== matlab function full_maneuver_single_veh/Fd_bkp/Virtual Vehicle Following/switch free flow/MATLAB Function ==
  data: h input; maxGap output; d0 input; vRef input; ev input; ehDot input; ea input; Kp parameter; Kd parameter; Ka parameter; Kdd parameter
function maxGap = followingGapThreshold(h, d0, vRef, ev, ehDot, ea, Kp, Kd, Ka, Kdd)

maxGap = h*vRef + d0 - 1/Kp*(Kd*ev + Kdd*ehDot + Ka*ea);

== matlab function full_maneuver_single_veh/Fd_bkp/Virtual Vehicle Following/switch min vel/MATLAB Function ==
  data: h input; maxGap output; d0 input; vRef input; ev input; ehDot input; ea input; Kp parameter; Kd parameter; Ka parameter; Kdd parameter
function maxGap = followingGapThreshold(h, d0, vRef, ev, ehDot, ea, Kp, Kd, Ka, Kdd)

maxGap = h*vRef + d0 - 1/Kp*(Kd*ev + Kdd*ehDot + Ka*ea);

== stateflow chart full_maneuver_single_veh/p1/ControlChoice ==
  state RegVehFoll
    entry:
    state = 0;
    during:
    u = regFollInput;
  state AdjForLaneChange
    during:
    %if ~xor(leaderInRange, vLeaderInRange)
    state = 1;
    u = min(regFollInput, virtualFollInput);
    %elseif vLeaderInRange
    %    state = 2;
    %    u = virtualFollInput;
    %else
    %    state = 3;
    %    u = regFollInput;
    %end
  (default) -> RegVehFoll
  AdjForLaneChange -> RegVehFoll : [~vLeaderAssigned]
  RegVehFoll -> AdjForLaneChange : [startAdj && vLeaderAssigned]
  data: startAdj input; vLeaderAssigned input; regFollInput input; u output; virtualFollInput input; state output

== matlab function full_maneuver_single_veh/p1/Find Leader/Subsystem/MATLAB Function ==
  data: ego input Bus: vehStatesBus; allVehicles input; leaderIdx output
function leaderIdx  = findLeader(ego, allVehicles)

nv = length(allVehicles);

leaderIdx = nv+1;

farAwayVehicle.X = ego.X + 10^4;
farAwayVehicle.Y = ego.Y;
farAwayVehicle.Xdot = ego.Xdot;
farAwayVehicle.u = 0;

leader = farAwayVehicle;
% For non lane changing vehicles, the leader is whoever is longitudinally
% closer and with any part of the body in the same lane.
% 1.8m (half lane) + 0.9m (half veh width)
for n = 1:nv
    if allVehicles(n).X>ego.X
        if abs(allVehicles(n).Y - ego.Y)<=2.7 && allVehicles(n).X<leader.X
            leaderIdx = n;
        end
    end
end

== matlab function full_maneuver_single_veh/p1/Platoon Gap Generation Management/assignExtraSpace ==
  data: strategy input; extraSpaceFlag output; posInPlatoon input; platoonState input
function extraSpaceFlag = assignExtraSpace(strategy, posInPlatoon, platoonState)

myState = platoonState(posInPlatoon);

%%% Single vehicle case %%%
if length(platoonState)==1 
    extraSpaceFlag = myState<5;
    return
end

%%% Platoon case %%%
switch strategy
    case {1, 2}
        if posInPlatoon == 1
            followerState = platoonState(posInPlatoon+1);
            extraSpaceFlag = myState<5 || followerState<6; %any(platoonState<5)
        elseif posInPlatoon == length(platoonState)
            leaderState = platoonState(posInPlatoon-1);
            extraSpaceFlag = leaderState>1 && myState<5;
        else
            leaderState = platoonState(posInPlatoon-1);
            followerState = platoonState(posInPlatoon+1);
            extraSpaceFlag = leaderState>1 && (myState<5 || followerState<6);
        end
%     case 2
%         if posInPlatoon == 1
%             extraSpaceFlag = true;
%         else
%             extraSpaceFlag = platoonState(posInPlatoon-1)>5;
%         end
    case 3
        if posInPlatoon == length(platoonState)
            extraSpaceFlag = myState<5 || platoonState(1)<5;%any(platoonState<5)
            % eventually try platoonState(end-1)<5
        else
           followerState = platoonState(posInPlatoon+1); 
           extraSpaceFlag = followerState>4 && (myState<5 || followerState<6);
        end 
    otherwise
        error('Unknown strategy')
end

== matlab function full_maneuver_single_veh/p1/Platoon Gap Generation Management/assignvirtualLeader ==
  data: strategy input; virtualLeaderFlag output; posInPlatoon input; platoonState input
function virtualLeaderFlag = assignVirtualLeader(strategy, posInPlatoon, platoonState)

myState = platoonState(posInPlatoon);

%%% Single vehicle case %%%
if length(platoonState)==1 
    virtualLeaderFlag = myState<5;
    return
end

%%% Platoon case %%%
switch strategy
    case {1, 2}
        if posInPlatoon == 1
            virtualLeaderFlag = myState<5;
        else
            leaderState = platoonState(posInPlatoon-1);
            virtualLeaderFlag = leaderState>3 && myState<5 ;
        end
    case 3
        if posInPlatoon == 1
           followerState = platoonState(posInPlatoon+1);
           virtualLeaderFlag = followerState>4 && (myState<5 || followerState<6);
        elseif posInPlatoon == length(platoonState)
            leaderState = platoonState(posInPlatoon-1);
            virtualLeaderFlag = myState<5 || leaderState<5;
            % first condition is redundant since leaderState won't change
            % if myState<5 - leaving it there for clarity and completeness
        else
           leaderState = platoonState(posInPlatoon-1); 
           followerState = platoonState(posInPlatoon+1);
           virtualLeaderFlag = followerState>4 && (myState<5 || leaderState<5);
        end 
    otherwise
        error('Unknown strategy')
end

== matlab function full_maneuver_single_veh/p1/Regular Vehicle Following/switch free flow/MATLAB Function ==
  data: h input; maxGap output; d0 input; vRef input; ev input; ehDot input; ea input; Kp parameter; Kd parameter; Ka parameter; Kdd parameter
function maxGap = followingGapThreshold(h, d0, vRef, ev, ehDot, ea, Kp, Kd, Ka, Kdd)

maxGap = h*vRef + d0 - 1/Kp*(Kd*ev + Kdd*ehDot + Ka*ea);

== matlab function full_maneuver_single_veh/Lo/Regular Vehicle Following/switch/MATLAB Function ==
  data: h input; maxGap output; d0 input; vRef input; ev input; ehDot input; ea input; Kp parameter; Kd parameter; Ka parameter; Kdd parameter
function maxGap = followingGapThreshold(h, d0, vRef, ev, ehDot, ea, Kp, Kd, Ka, Kdd)

maxGap = h*vRef + d0 - 1/Kp*(Kd*ev + Kdd*ehDot + Ka*ea);

== matlab function full_maneuver_single_veh/p1/Virtual Follower Manager/determineVirtualFollower ==
  data: nVehicles input; posInPlatoon input; lcStrategy input; virtualFollowerIdx output
function virtualFollowerIdx  = ...
    determineVirtualFollower(nVehicles, posInPlatoon, lcStrategy)

% Important assumption:
% The array of vehicles is ordered as [Ld, Fd, Lo, p1, ..., pN, Fo]

% To consider: would it be more organized to have two vehicle arrays (one 
% for each lane)?

switch lcStrategy
    case {1, 2} % synchronous, leader changes first
        virtualFollowerIdx = 2;
    case 3 % last veh changes first
        if posInPlatoon == nVehicles-4
            virtualFollowerIdx = 2;
        else
            virtualFollowerIdx = 3 + (posInPlatoon + 1);
        end
    otherwise
        error('[determineVirtualFollower in Simulink model] Unknown lane changing strategy]')
end

end

== matlab function full_maneuver_single_veh/p1/Virtual Leader Manager/determineVirtualLeader ==
  data: nVehicles input; lcFlag input; lcDone input; virtualLeaderIdx output; posInPlatoon input; lcStrategy input
function virtualLeaderIdx  = ...
    determineVirtualLeader(nVehicles, lcFlag, lcDone, posInPlatoon, lcStrategy)

% Important assumption:
% The array of vehicles is ordered as [Ld, Fd, Lo, p1, ..., pN, Fo]

% To consider: would it be more organized to have two vehicle arrays (one 
% for each lane)?

if ~lcFlag% gap generating vehicle
    virtualLeaderIdx = nVehicles-1; % last platoon vehicle
    
else % lane changing vehicle
    switch lcStrategy
        case {1, 2} % synchronous, leader changes first
            if posInPlatoon == 1
                virtualLeaderIdx = 1;
            else
                virtualLeaderIdx = 3 + (posInPlatoon - 1);
            end
            
        case 3 % last veh changes first
            if ~lcDone
                virtualLeaderIdx = 1;
            else
                if posInPlatoon == 1
                    virtualLeaderIdx = 1;
                else
                    virtualLeaderIdx = 3 + (posInPlatoon - 1);
                end
            end
            
        otherwise
            error('[determineVirtualLeader in Simulink model] Unknown lane changing strategy]')
    end
end

end

== stateflow chart full_maneuver_single_veh/Fd/ControlChoice ==
  state RegVehFoll
    entry:
    state = 0;
    during:
    u = regFollInput;
  state AdjForLaneChange
    during:
    %if ~xor(leaderInRange, vLeaderInRange)
    state = 1;
    u = min(regFollInput, virtualFollInput);
    %elseif vLeaderInRange
    %    state = 2;
    %    u = virtualFollInput;
    %else
    %    state = 3;
    %    u = regFollInput;
    %end
  (default) -> RegVehFoll
  AdjForLaneChange -> RegVehFoll : [~vLeaderAssigned]
  RegVehFoll -> AdjForLaneChange : [startAdj && vLeaderAssigned]
  data: startAdj input; vLeaderAssigned input; regFollInput input; u output; virtualFollInput input; state output

== matlab function full_maneuver_single_veh/Fd/Find Leader/Subsystem/MATLAB Function ==
  data: ego input Bus: vehStatesBus; allVehicles input; leaderIdx output
function leaderIdx  = findLeader(ego, allVehicles)

nv = length(allVehicles);

leaderIdx = nv+1;

farAwayVehicle.X = ego.X + 10^4;
farAwayVehicle.Y = ego.Y;
farAwayVehicle.Xdot = ego.Xdot;
farAwayVehicle.u = 0;

leader = farAwayVehicle;
% For non lane changing vehicles, the leader is whoever is longitudinally
% closer and with any part of the body in the same lane.
% 1.8m (half lane) + 0.9m (half veh width)
for n = 1:nv
    if allVehicles(n).X>ego.X
        if abs(allVehicles(n).Y - ego.Y)<=2.7 && allVehicles(n).X<leader.X
            leaderIdx = n;
        end
    end
end

== matlab function full_maneuver_single_veh/p1/Virtual Vehicle Following/switch min vel/MATLAB Function ==
  data: h input; maxGap output; d0 input; vRef input; ev input; ehDot input; ea input; Kp parameter; Kd parameter; Ka parameter; Kdd parameter
function maxGap = followingGapThreshold(h, d0, vRef, ev, ehDot, ea, Kp, Kd, Ka, Kdd)

maxGap = h*vRef + d0 - 1/Kp*(Kd*ev + Kdd*ehDot + Ka*ea);

== matlab function full_maneuver_single_veh/Ld/findLeader/Subsystem/MATLAB Function ==
  data: ego input Bus: vehStatesBus; allVehicles input; leaderIdx output
function leaderIdx  = findLeader(ego, allVehicles)

nv = length(allVehicles);

leaderIdx = nv+1;

farAwayVehicle.X = ego.X + 10^4;
farAwayVehicle.Y = ego.Y;
farAwayVehicle.Xdot = ego.Xdot;
farAwayVehicle.u = 0;

leader = farAwayVehicle;
% For non lane changing vehicles, the leader is whoever is longitudinally
% closer and with any part of the body in the same lane.
% 1.8m (half lane) + 0.9m (half veh width)
for n = 1:nv
    if allVehicles(n).X>ego.X
        if abs(allVehicles(n).Y - ego.Y)<=2.7 && allVehicles(n).X<leader.X
            leaderIdx = n;
        end
    end
end

== matlab function full_maneuver_single_veh/Lo/findLeader/Subsystem/MATLAB Function ==
  data: ego input Bus: vehStatesBus; allVehicles input; leaderIdx output
function leaderIdx  = findLeader(ego, allVehicles)

nv = length(allVehicles);

leaderIdx = nv+1;

farAwayVehicle.X = ego.X + 10^4;
farAwayVehicle.Y = ego.Y;
farAwayVehicle.Xdot = ego.Xdot;
farAwayVehicle.u = 0;

leader = farAwayVehicle;
% For non lane changing vehicles, the leader is whoever is longitudinally
% closer and with any part of the body in the same lane.
% 1.8m (half lane) + 0.9m (half veh width)
for n = 1:nv
    if allVehicles(n).X>ego.X
        if abs(allVehicles(n).Y - ego.Y)<=2.7 && allVehicles(n).X<leader.X
            leaderIdx = n;
        end
    end
end
